simulink model "Reaching"  (R2024b)
settings: Solver=FixedStepDiscrete  StartTime=0.0  StopTime=inf  FixedStep=0.001  RelTol=1e-3
undefined symbols (not defined in the file): get
libraries: PhanTorque_3Dof_Library_64Bits x1, vrlib x1
settings Model: Creator=carlos.aldana  LastModifiedBy=elima
settings SolverCC: AlgebraicLoopSolver=TrustRegion
settings DataIOCC: LimitDataPoints=on  SaveFormat=Array  ReturnWorkspaceOutputs=off
settings OptimizationCC: BlockReduction=off  BooleanDataType=off  LifeSpan=inf
settings DebuggingCC: SaveWithParameterizedLinksMsg=none  UnderspecifiedInitializationDetection=Classic  MergeDetectMultiDrivingBlocksExec=none  SignalResolutionControl=TryResolveAllWithWarning  UnconnectedInputMsg=warning  UnconnectedOutputMsg=warning  UnconnectedLineMsg=warning  AllowSymbolicDim=off  SFUnexpectedBacktrackingDiag=warning  SFNoUnconditionalDefaultTransitionDiag=warning  SFExecutionAtInitializationDiag=none  ArithmeticOperatorsInVariantConditions=warning
settings HardwareCC: ProdBitPerPointer=32  ProdBitPerSizeT=32  ProdBitPerPtrDiffT=32  ProdLargestAtomicFloat=None  ProdIntDivRoundTo=Undefined  ProdEndianess=Unspecified  ProdWordSize=32  ProdHWDeviceType=32-bit Generic  TargetUnknown=on
settings ModelReferenceCC: EnableRefExpFcnMdlSchedulingChecks=on  PropagateSignalLabelsOutOfModel=off
settings SFSimCC: SimUseLocalCustomCode=off  CustomCodeUndefinedFunction=UseInterfaceOnly
settings RTWCC: RTWUseLocalCustomCode=off  GPUComputeCapability=3.5  DLArmComputeVersion=19.05
settings CodeAppCC: StateflowObjectComments=on
settings GRTTargetCC: TargetLangStandard=C89/C90 (ANSI)
settings ConfigComp: CovMetricSettings=dw  CovSaveCumulativeToWorkspaceVar=on  CovSaveSingleToWorkspaceVar=on  CovExternalEMLEnable=off  CovSFcnEnable=off

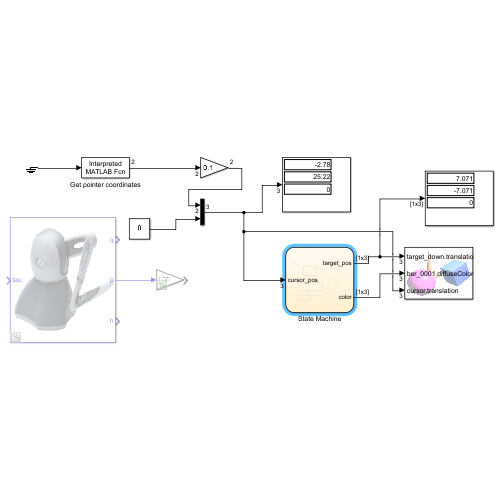
[thumbnail: Simulink's stored preview of the top-level diagram]
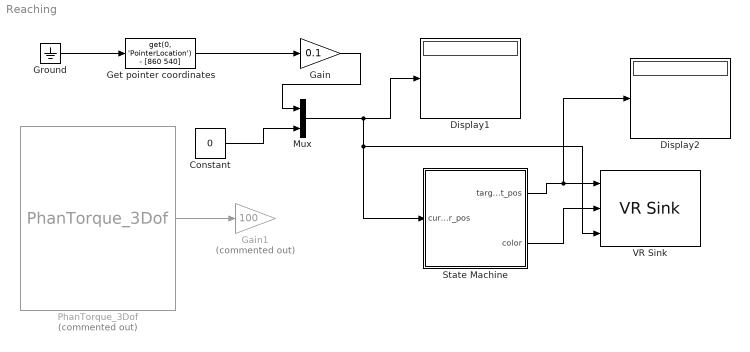
== system Reaching ==
  Constant : Constant  Value=0
  Display1 : Display
  Display2 : Display
  Gain : Gain  Gain=0.1
  Gain1 : Gain  Commented=on  Gain=100
  Get pointer coordinates : MATLABFcn  MATLABFcn=get(0, 'PointerLocation') - [860 540]  OutputDimensions=2
  Ground : Ground
  Mux : Mux  Inputs=2
  PhanTorque_3Dof : PhanTorque_3Dof_Library_64Bits/PhanTorque_3Dof  Commented=on  Haptic_Name='Default Device'
  State Machine : Stateflow chart  TreatAsAtomicUnit=on
  VR Sink : vrlib/VR Sink  InstantiateOnLoad=on  SampleTime=0.1  ViewEnable=on  RemoteChange=off  RemoteView=off  FieldsWritten=target_down.translation.3.1.1.double#ber_0001.diffuseColor.3.1.1.double#cursor.translation.3.1.1.double  WorldFileName=VR_centerAndTarget.wrl  AutoView=off  VideoDimensions=[]  AllowVariableSize=off
  wires:
  Get pointer coordinates/1 -> Gain/1
  Ground/1 -> Get pointer coordinates/1
  State Machine/1(target_pos) -> Display2/1, VR Sink/1
  State Machine/2(color) -> VR Sink/2
  Gain/1 -> Mux/1
  Constant/1 -> Mux/2
  PhanTorque_3Dof/2 -> Gain1/1
  Mux/1 -> VR Sink/3, State Machine/1(cursor_pos), Display1/1

== stateflow chart Reaching/State Machine ==
  settings: updateMethod=DISCRETE
  state Initializing
    entry:
    color = [0, 1, 1];
    target_pos = [0, 0, 0];
  state New_target
    entry:
    angle = counter * (pi/4);
    target_pos = [radius * cos(angle), radius * sin(angle), 0];
  state Finish
    entry:
    color = [0, 1, 0];
  state Finish2
    entry:
    color = [0, 1, 1];
  (default) -> Initializing : {counter = 0}
  Finish -> Initializing [order 1] : [temporalCount(sec) >=  1 && counter < 7]{counter = counter + 1}
  Initializing -> New_target : [temporalCount(sec) >= 2 && double(norm(cursor_pos - target_pos)) < 1.0]
  New_target -> Finish : [double(norm(cursor_pos - target_pos)) < 1.0]
  Finish2 -> Finish : [double(norm(cursor_pos - target_pos)) < 1.0]
  Finish -> Finish2 [order 2] : [double(norm(cursor_pos - target_pos)) > 1.0]
  data: target_pos output double size=[1 3]; color output double size=[1 3]; cursor_pos input size=[1 3]; counter local; radius constant double =10; angle local double
